simulink model "ESE5050_HW9_simulinkModel"  (R2024b)
settings: Solver=ode3  StartTime=0.0  StopTime=50  FixedStep=0.01  RelTol=1e-3
settings Model: Creator=hesha  LastModifiedBy=hesha

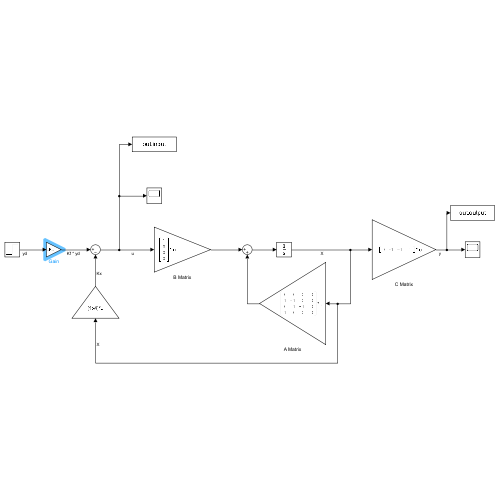
[thumbnail: Simulink's stored preview of the top-level diagram]
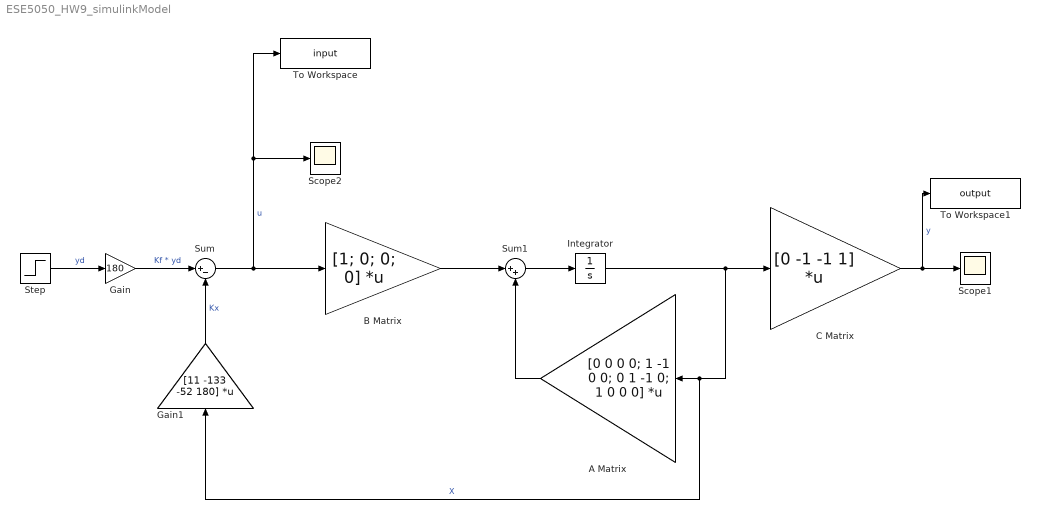
== system ESE5050_HW9_simulinkModel ==
  A Matrix : Gain  Gain=[0 0 0 0; 1 -1 0 0; 0 1 -1 0; 1 0 0 0]  Multiplication=Matrix(K*u)
  B Matrix : Gain  Gain=[1; 0; 0; 0]  Multiplication=Matrix(K*u)
  C Matrix : Gain  Gain=[0 -1 -1 1]  Multiplication=Matrix(K*u)
  Gain : Gain  Gain=180
  Gain1 : Gain  Gain=[11 -133 -52 180]  Multiplication=Matrix(K*u)
  Integrator : Integrator
  Scope1 : Scope
  Scope2 : Scope
  Step : Step  SampleTime=0
  Sum : Sum  Inputs=|+-
  Sum1 : Sum  Inputs=|++
  To Workspace : ToWorkspace  VariableName=input  SampleTime=-1
  To Workspace1 : ToWorkspace  VariableName=output  SampleTime=-1
  wires:
  Step/1 -> Gain/1  "yd"
  Gain/1 -> Sum/1  "Kf * yd"
  Gain1/1 -> Sum/2  "Kx"
  Sum1/1 -> Integrator/1
  C Matrix/1 -> Scope1/1, To Workspace1/1  "y"
  A Matrix/1 -> Sum1/2
  B Matrix/1 -> Sum1/1
  Integrator/1 -> A Matrix/1, Gain1/1, C Matrix/1  "X"
  Sum/1 -> Scope2/1, To Workspace/1, B Matrix/1  "u"
